simulink model "EEGRecorder"  (R2019a)
settings: Solver=VariableStepAuto  StartTime=0.0  StopTime=inf  RelTol=1e-3
undefined symbols (not defined in the file): daq
libraries: dspnetwork x2, daqlib x1
settings Model: Creator=Kusunoki  LastModifiedBy=Owner

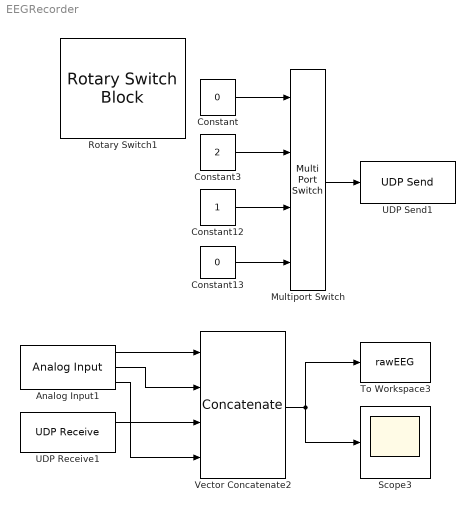
== system EEGRecorder ==
  Analog Input1 : daqlib/Analog Input  DeviceMenu=ni Dev1 (USB-6000)  Device=ni Dev1 (USB-6000)  ObjConstructor=daq.createSession('ni')  NChannelsSelected=2  Channels=1$ai0$$Dev1$1$1$1$1$#1$ai1$$Dev1$1$1$1$1$#0$ai2$$Dev1$1$1$1$1$#0$ai3$$Dev1$1$1$1$1$#0$ai4$$Dev1$1$1$1$1$#0$ai5$$Dev1$1$1$1$1$#0$ai6$$Dev1$1$1$1$1$#0$ai7$$Dev1$1$1$1$1$#  NPorts=1 per channel  SampleRate=2000  ActualRate=2000  ScansPerTrigger=200  OutputTimestamp=on  AcqMode=0  NumFrameBuffer=100  OutputTriggertime=off
      settings: SourceProductName=Data Acquisition Toolbox  SourceProductBaseCode=DA
  Constant : Constant  Value=0
  Constant12 : Constant
  Constant13 : Constant  Value=0
  Constant3 : Constant  Value=2
  Multiport Switch : MultiPortSwitch  DataPortOrder=Specify indices  DataPortIndices={2,1,0}
  Rotary Switch1 : RotarySwitchBlock
      settings: Values={{'0 : nothing', '1 : stick', '2 : ball'}, [0 1 2]}
  Scope3 : Scope
  To Workspace3 : ToWorkspace  VariableName=rawEEG  SampleTime=-1
  UDP Receive1 : dspnetwork/UDP Receive  localURL='0.0.0.0'  localPort=25000  remoteURL='0.0.0.0'  remotePort=-1  recvBufferSize=8192  dims=200  signalDatatype=double  isComplex=off  isVarSize=off  showBlockingTime=off  blockingTime=0  sampletime=0.0005  blockPlatform=[]
      settings: SourceProductName=Simulink
  UDP Send1 : dspnetwork/UDP Send  remoteURL='127.0.0.1'  remotePort=25000  localURL='0.0.0.0'  localPortSource=Automatically determine  localPort=-1  sampletime=-1  blockPlatform=[]  separateLengthPort=0
      settings: SourceProductName=Simulink
  Vector Concatenate2 : Concatenate  NumInputs=4  Mode=Multidimensional array  ConcatenateDimension=2
  wires:
  Analog Input1/1 -> Vector Concatenate2/1
  UDP Receive1/1 -> Vector Concatenate2/3
  Vector Concatenate2/1 -> Scope3/1, To Workspace3/1
  Constant13/1 -> Multiport Switch/4
  Constant3/1 -> Multiport Switch/2
  Multiport Switch/1 -> UDP Send1/1
  Constant12/1 -> Multiport Switch/3
  Constant/1 -> Multiport Switch/1
  Analog Input1/2 -> Vector Concatenate2/2
  Analog Input1/3 -> Vector Concatenate2/4
